simulink model "tcp_server_2017b"  (R2017b)
settings: Solver=ode3  StartTime=0.0  StopTime=10  FixedStep=0.1  RelTol=1e-3
settings Model: ExtModeArmWhenConnect=off  Creator=Zhang Lei  LastModifiedBy=yaozhong.zhang
settings DataIOCC: LimitDataPoints=on  SaveFormat=Array  SignalLoggingSaveFormat=ModelDataLogs
settings OptimizationCC: BlockReduction=off  BooleanDataType=off  LifeSpan=inf
settings DebuggingCC: SaveWithParameterizedLinksMsg=none  UnderspecifiedInitializationDetection=Classic  MergeDetectMultiDrivingBlocksExec=none  SignalResolutionControl=TryResolveAllWithWarning  MultiTaskDSMMsg=warning  MultiTaskCondExecSysMsg=none  SFUnexpectedBacktrackingDiag=warning  SFNoUnconditionalDefaultTransitionDiag=warning  SFExecutionAtInitializationDiag=none
settings HardwareCC: ProdBitPerPointer=32  ProdBitPerSizeT=32  ProdBitPerPtrDiffT=32  ProdLargestAtomicFloat=None  ProdIntDivRoundTo=Undefined  ProdEndianess=Unspecified  ProdWordSize=32  ProdHWDeviceType=32-bit Generic  TargetUnknown=on
settings ModelReferenceCC: PropagateSignalLabelsOutOfModel=off
settings CodeAppCC: StateflowObjectComments=on
settings GRTTargetCC: TargetLangStandard=C89/C90 (ANSI)  GeneratePreprocessorConditionals=Disable all
settings ConfigComp: CovMetricSettings=dw  CovHtmlReporting=on  CovSaveCumulativeToWorkspaceVar=on  CovSaveSingleToWorkspaceVar=on  CovExternalEMLEnable=off

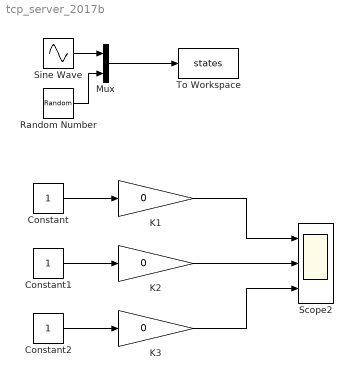
== system tcp_server_2017b ==
  Constant : Constant
  Constant1 : Constant
  Constant2 : Constant
  K1 : Gain  Gain=0
  K2 : Gain  Gain=0
  K3 : Gain  Gain=0
  Mux : Mux  Inputs=2
  Random Number : RandomNumber  SampleTime=0.1
  Scope2 : Scope  NumInputPorts=3
  Sine Wave : Sin  SampleTime=0
  To Workspace : ToWorkspace  VariableName=states  SaveFormat=Timeseries  SampleTime=-1
  wires:
  Constant/1 -> K1/1
  K1/1 -> Scope2/1
  Sine Wave/1 -> Mux/1
  Mux/1 -> To Workspace/1
  Random Number/1 -> Mux/2
  Constant1/1 -> K2/1
  K2/1 -> Scope2/2
  Constant2/1 -> K3/1
  K3/1 -> Scope2/3
